simulink model "MAS_Full_State_AS_2021a"  (R2021a)
settings: Solver=VariableStepAuto  StartTime=0.0  StopTime=50  RelTol=1e-3
libraries: cstblocks x15
settings Model: Creator=lenovo  LastModifiedBy=lenovo

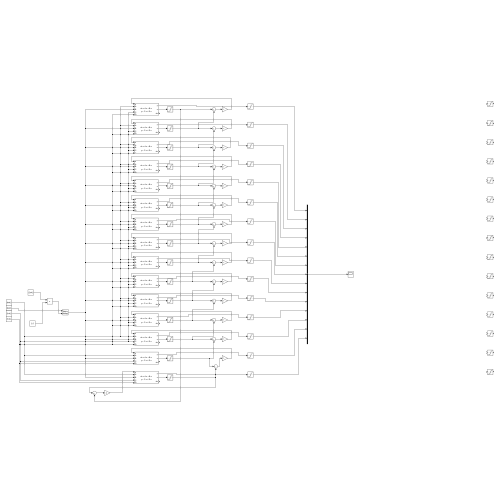
[thumbnail: Simulink's stored preview of the top-level diagram]
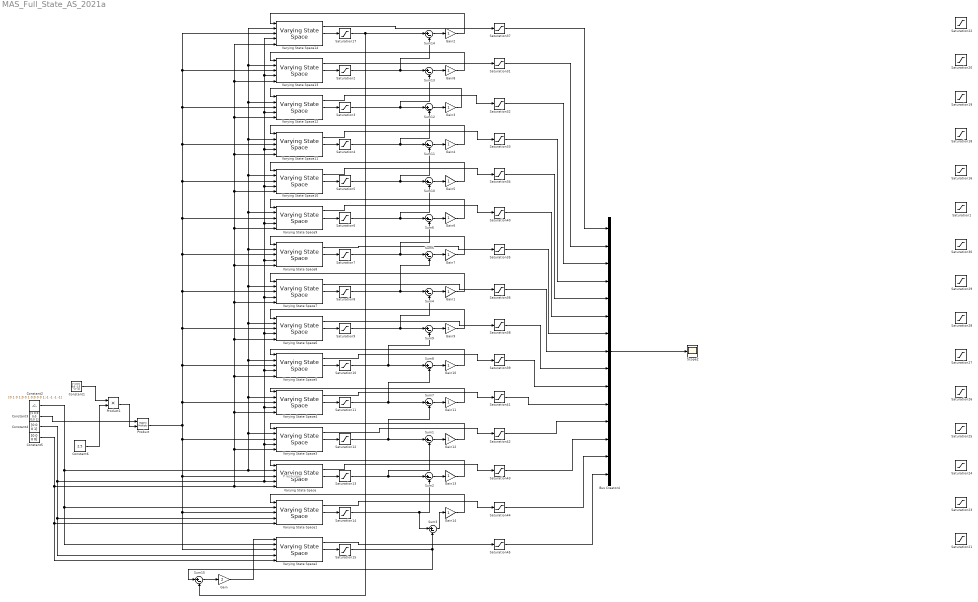
== system MAS_Full_State_AS_2021a ==
  note: P resburger
  Bus Creator4 : BusCreator  Inputs=15
  Constant1 : Constant  Value=[-1 0 0 0;0 -1.5 -2 -1]
  Constant2 : Constant  Value=[0 1 0 1;0 0 1 0;0 0 0 1;-1 -1 -1 -1]
  Constant3 : Constant  Value=[1 0;0 0;0 0;0 1]
  Constant4 : Constant  Value=[0 0 0 1]  VectorParams1D=off
  Constant5 : Constant  Value=[0 0 0 0]  VectorParams1D=off
  Constant6 : Constant  Value=2.5  VectorParams1D=off
  Gain : Gain  Gain=2
  Gain{1..14} (14 alike) : Gain
  Product : Product  Multiplication=Matrix(*)
  Product1 : Product
  Saturation{1,16,18..45} (30 alike) : Saturate  UpperLimit=1  LowerLimit=-1
  Saturation{2..15,17} (15 alike) : Saturate  UpperLimit=0.05  LowerLimit=-0.05
  Scope2 : Scope
  Sum{1..15} (15 alike) : Sum  Inputs=|+-
  Varying State Space{,1,3..14} (14 alike) : cstblocks/Linear Parameter Varying/Varying State Space  x0=0  xNames=''  OutputX=on  OutputDX=on
  Varying State Space2 : cstblocks/Linear Parameter Varying/Varying State Space  x0=[1;0;0;0]  xNames=''  OutputX=on  OutputDX=on
  wires:
  Gain/1 -> Varying State Space2/1
  Constant3/1 -> Product/1
  Bus Creator4/1 -> Scope2/1
  Product1/1 -> Product/2
  Constant1/1 -> Product1/1
  Constant5/1 -> Varying State Space2/5, Varying State Space1/5, Varying State Space3/5, Varying State Space4/5, Varying State Space5/5, Varying State Space7/5, Varying State Space8/5, Varying State Space9/5, Varying State Space10/5, Varying State Space11/5, Varying State Space13/5, Varying State Space14/5, Varying State Space12/5, Varying State Space6/5, Varying State Space/5
  Product/1 -> Varying State Space3/3, Varying State Space2/3, Varying State Space1/3, Varying State Space/3, Varying State Space7/3, Varying State Space8/3, Varying State Space9/3, Varying State Space10/3, Varying State Space11/3, Varying State Space12/3, Varying State Space14/3, Varying State Space13/3, Varying State Space6/3, Varying State Space5/3, Varying State Space4/3
  Constant4/1 -> Varying State Space2/4, Varying State Space1/4, Varying State Space9/4, Varying State Space14/4, Varying State Space13/4, Varying State Space12/4, Varying State Space11/4, Varying State Space10/4, Varying State Space8/4, Varying State Space7/4, Varying State Space6/4, Varying State Space5/4, Varying State Space4/4, Varying State Space3/4, Varying State Space/4
  Constant2/1 -> Varying State Space2/2, Varying State Space1/2, Varying State Space3/2, Varying State Space4/2, Varying State Space5/2, Varying State Space7/2, Varying State Space8/2, Varying State Space9/2, Varying State Space10/2, Varying State Space11/2, Varying State Space12/2, Varying State Space14/2, Varying State Space13/2, Varying State Space6/2, Varying State Space/2
  Constant6/1 -> Product1/2
  Varying State Space11/2 -> Saturation4/1
  Varying State Space2/2 -> Saturation15/1
  Varying State Space1/2 -> Saturation14/1
  Varying State Space/2 -> Saturation13/1
  Varying State Space3/2 -> Saturation12/1
  Varying State Space4/2 -> Saturation11/1
  Varying State Space14/2 -> Saturation17/1
  Varying State Space13/2 -> Saturation2/1
  Varying State Space12/2 -> Saturation3/1
  Varying State Space10/2 -> Saturation5/1
  Varying State Space9/2 -> Saturation6/1
  Varying State Space8/2 -> Saturation7/1
  Varying State Space7/2 -> Saturation8/1
  Varying State Space6/2 -> Saturation9/1
  Varying State Space5/2 -> Saturation10/1
  Saturation15/1 -> Sum3/2, Sum15/1
  Saturation14/1 -> Sum3/1, Sum2/2
  Saturation13/1 -> Sum2/1, Sum1/2
  Saturation12/1 -> Sum1/1, Sum7/2
  Saturation11/1 -> Sum8/2, Sum7/1
  Saturation10/1 -> Sum8/1, Sum9/2
  Saturation9/1 -> Sum9/1, Sum4/2
  Saturation8/1 -> Sum4/1, Sum5/2
  Saturation7/1 -> Sum5/1, Sum6/2
  Saturation6/1 -> Sum6/1, Sum10/2
  Saturation5/1 -> Sum10/1, Sum11/2
  Saturation4/1 -> Sum12/2, Sum11/1
  Saturation3/1 -> Sum12/1, Sum13/2
  Saturation2/1 -> Sum13/1, Sum14/2
  Saturation17/1 -> Sum15/2, Sum14/1
  Varying State Space14/1 -> Saturation37/1
  Varying State Space13/1 -> Saturation31/1
  Varying State Space12/1 -> Saturation32/1
  Varying State Space11/1 -> Saturation33/1
  Varying State Space10/1 -> Saturation34/1
  Varying State Space9/1 -> Saturation40/1
  Varying State Space8/1 -> Saturation35/1
  Varying State Space7/1 -> Saturation36/1
  Varying State Space6/1 -> Saturation38/1
  Varying State Space5/1 -> Saturation39/1
  Varying State Space4/1 -> Saturation41/1
  Varying State Space3/1 -> Saturation42/1
  Varying State Space/1 -> Saturation43/1
  Varying State Space1/1 -> Saturation44/1
  Varying State Space2/1 -> Saturation45/1
  Saturation45/1 -> Bus Creator4/15
  Saturation44/1 -> Bus Creator4/14
  Saturation43/1 -> Bus Creator4/13
  Saturation42/1 -> Bus Creator4/12
  Saturation41/1 -> Bus Creator4/11
  Saturation39/1 -> Bus Creator4/10
  Saturation38/1 -> Bus Creator4/9
  Saturation36/1 -> Bus Creator4/8
  Saturation35/1 -> Bus Creator4/7
  Saturation40/1 -> Bus Creator4/6
  Saturation34/1 -> Bus Creator4/5
  Saturation33/1 -> Bus Creator4/4
  Saturation32/1 -> Bus Creator4/3
  Saturation31/1 -> Bus Creator4/2
  Saturation37/1 -> Bus Creator4/1
  Sum15/1 -> Gain/1
  Sum14/1 -> Gain2/1
  Gain2/1 -> Varying State Space14/1
  Sum3/1 -> Gain14/1
  Sum2/1 -> Gain13/1
  Sum1/1 -> Gain12/1
  Sum13/1 -> Gain8/1
  Gain8/1 -> Varying State Space13/1
  Sum12/1 -> Gain3/1
  Gain3/1 -> Varying State Space12/1
  Sum11/1 -> Gain4/1
  Gain4/1 -> Varying State Space11/1
  Sum10/1 -> Gain5/1
  Gain5/1 -> Varying State Space10/1
  Sum6/1 -> Gain6/1
  Gain6/1 -> Varying State Space9/1
  Gain7/1 -> Varying State Space8/1
  Sum5/1 -> Gain7/1
  Sum4/1 -> Gain1/1
  Gain1/1 -> Varying State Space7/1
  Sum9/1 -> Gain9/1
  Gain9/1 -> Varying State Space6/1
  Gain10/1 -> Varying State Space5/1
  Sum8/1 -> Gain10/1
  Sum7/1 -> Gain11/1
  Gain11/1 -> Varying State Space4/1
  Gain12/1 -> Varying State Space3/1
  Gain13/1 -> Varying State Space/1
  Gain14/1 -> Varying State Space1/1
